simulink model "lab2"  (R2021a)
settings: Solver=VariableStepAuto  StartTime=0.0  StopTime=10.0  MaxStep=1e-6  RelTol=1e-3
settings Model: Creator=Sosagayoo  LastModifiedBy=Sosagayoo

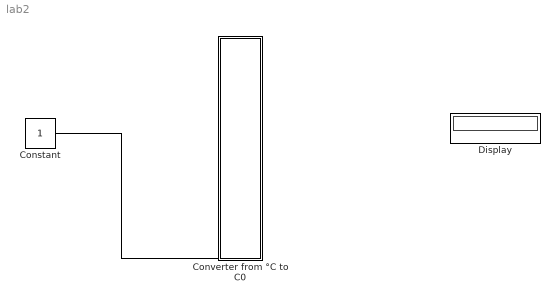
== system lab2 ==
  Constant : Constant
  Converter from °C to C0 : Subsystem
  Display : Display
  wires:
  Constant/1 -> ?
  ? -> Display/1

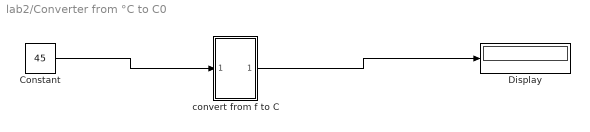
== system lab2/Converter from °C to C0 ==
  Constant : Constant  Value=45
  Display : Display
  convert from f to C : Subsystem
  wires:
  convert from f to C/1(Out1) -> Display/1
  Constant/1 -> convert from f to C/1(In1)

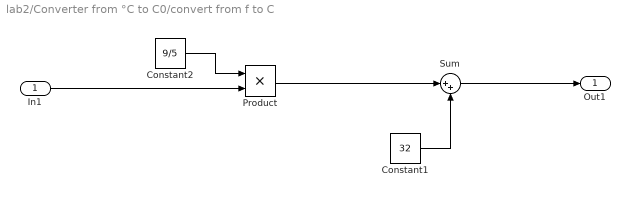
== system lab2/Converter from °C to C0/convert from f to C ==
  In1 : Inport
  Constant1 : Constant  Value=32
  Constant2 : Constant  Value=9/5
  Product : Product
  Sum : Sum  Inputs=|++
  Out1 : Outport
  wires:
  Product/1 -> Sum/1
  Constant1/1 -> Sum/2
  Sum/1 -> Out1/1
  Constant2/1 -> Product/1
  In1/1 -> Product/2
